simulink model "wurfwettesim"  (R2025b)
settings: Solver=VariableStepAuto  StartTime=0.0  StopTime=10.0  RelTol=1e-3
values from neighbouring files (symbols this model uses):
  h0i = [x0;-0.1*x0^2+Koerpergr]    [wurfwettefunc.m]
  v0i = v0*[cosd(alpha);sind(alpha)]    [wurfwettefunc.m]
libraries: simulink x1
settings Model: Creator=ssokolov  LastModifiedBy=ssokolov
settings DataIOCC: OutputSaveName=xy

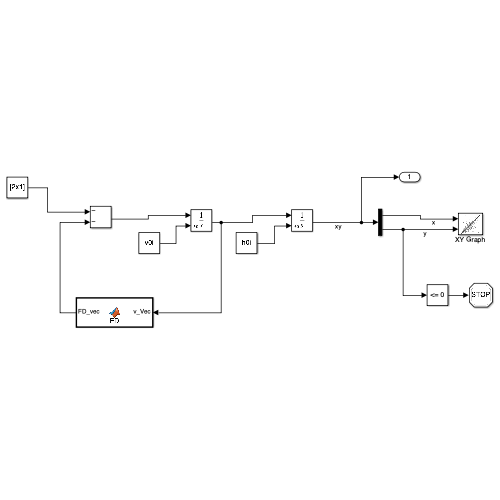
[thumbnail: Simulink's stored preview of the top-level diagram]
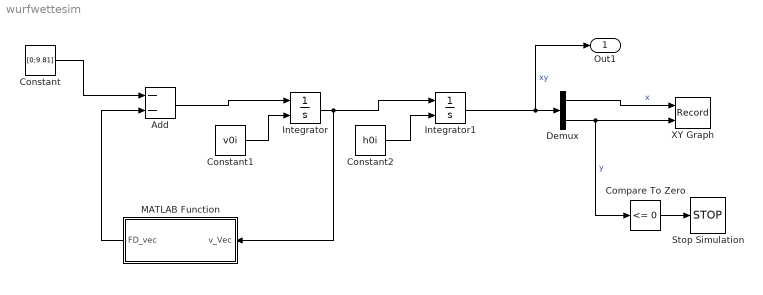
== system wurfwettesim ==
  Add : Sum  Inputs=--
  Compare To Zero : simulink/Logic and Bit Operations/Compare To Zero  relop=<=  OutDataTypeStr=boolean
  Constant : Constant  Value=[0;9.81]
  Constant1 : Constant  Value=v0i
  Constant2 : Constant  Value=h0i
  Demux : Demux  Outputs=2
  Integrator : Integrator  InitialConditionSource=external
  Integrator1 : Integrator  InitialConditionSource=external
  MATLAB Function : MATLAB Function  TreatAsAtomicUnit=on
  Stop Simulation : Stop
  XY Graph : Record  NumPorts=2.0  FileSettingsInternal="{\"entries\":[{\"content\":{\"excelSettings\":{\"content\":{},\"type\":\"Streamout.ExcelSettings\"},\"parquetSettings\":{\"content\":{},\"type\":\"Streamout.ParquetSettings\"}},\"type\":\"Streamout.FileSettingStorage\",\"uuid\":\"\"}],\"packageUris\":[\"http:\\/\\/schema.mathworks.com\\/mf0\\/streamout_blocks\\/R2020a\"],\"version\":\"1.0\"}"  FrameSettings=[0, 0]  Layout=[1 1]  SignalsInternal="{\"entries\":[{\"content\":{\"signals\":[{\"content\":{\"blockPath\":[],\"dimensions\":[1,1],\"domain\":\"\",\"lineColor\":\"#a2142f\",\"plots\":[ 1 ],\"port\":1,\"sid\":[\"\"],\"signalID\":1,\"signalName\":\"x\"},\"type\":\"RecordBlkView.Signal\",\"uuid\":\"\"},{\"content\":{\"blockPath\":[],\"dimensions\":[1,1],\"domain\":\"\",\"lineColor\":\"#139fff\",\"plots\":[ 1 ],\"port\":2,\"sid\":[\"\"],\"signalID\":2,\"signalName\":\"y\"},\"type\":\"RecordBlkView.Signal\",\"uuid\":\"\"}]},\"type\":\"RecordBlkView.InputSignals\",\"uuid\":\"\"}],\"packageUris\":[\"http:\\/\\/schema.mathworks.com\\/mf0\\/streamout_blocks\\/R2020a\"],\"version\":\"1.0\"}"  VisualizationBindings="{\"xyplotplugin\":{\"info\":[{\"series\":[{\"bindingParametersList\":[{\"parameter\":\"X-Axis\",\"signalID\":1,\"signalName\":\"x\"},{\"parameter\":\"Y-Axis\",\"signalID\":2,\"signalName\":\"y\"}],\"seriesID\":0}],\"subplotID\":1}]}}"  CompatibilityTag=XY
  Out1 : Outport
  wires:
  Constant/1 -> Add/1
  Add/1 -> Integrator/1
  Integrator/1 -> MATLAB Function/1(v_Vec), Integrator1/1
  Constant1/1 -> Integrator/2
  Constant2/1 -> Integrator1/2
  MATLAB Function/1(FD_vec) -> Add/2
  Demux/2 -> Compare To Zero/1, XY Graph/2  "y"
  Integrator1/1 -> Out1/1, Demux/1  "xy"
  Demux/1 -> XY Graph/1  "x"
  Compare To Zero/1 -> Stop Simulation/1

== matlab function wurfwettesim/MATLAB Function ==
  data: v_Vec input; FD_vec output
function FD_vec = FD(v_Vec)
%Constanten definieren
m=0.75;
d=0.24;
A=d^2*pi/4;
rho=1.225;
cw=0.45;

%Ausgang berechnen - FD/m (für DGL)
FD_vec = 1./(2*m)*rho*cw*A.*v_Vec.*abs(v_Vec);
